simulink model "kinematic_steering"  (R2023b)
settings: Solver=VariableStepAuto  StartTime=0.0  StopTime=10.0  RelTol=1e-3
undefined symbols (not defined in the file or in its folder): static_toe_front, static_toe_rear, steering_rack_to_axis_distance
libraries: simulink_extras x7, vehdynlibsteering x1
settings Model: Creator=bglen  LastModifiedBy=bglen

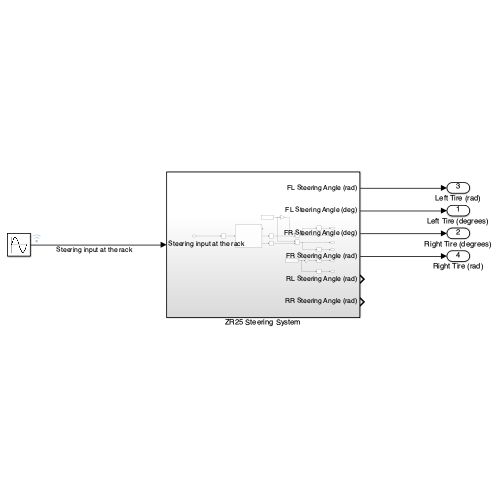
[thumbnail: Simulink's stored preview of the top-level diagram]
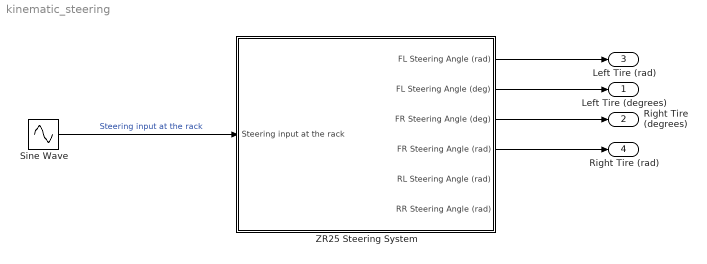
== system kinematic_steering ==
  Sine Wave : Sin  Amplitude=90  SampleTime=0
  ZR25 Steering System : Subsystem
  Left Tire (degrees) : Outport
  Right Tire (degrees) : Outport  Port=2
  Left Tire (rad) : Outport  Port=3
  Right Tire (rad) : Outport  Port=4
  wires:
  Sine Wave/1 -> ZR25 Steering System/1(Steering input at the rack)  "Steering input at the rack"
  ZR25 Steering System/1(FL Steering Angle (rad)) -> Left Tire (rad)/1
  ZR25 Steering System/2(FL Steering Angle (deg)) -> Left Tire (degrees)/1
  ZR25 Steering System/3(FR Steering Angle (deg)) -> Right Tire (degrees)/1
  ZR25 Steering System/4(FR Steering Angle (rad)) -> Right Tire (rad)/1

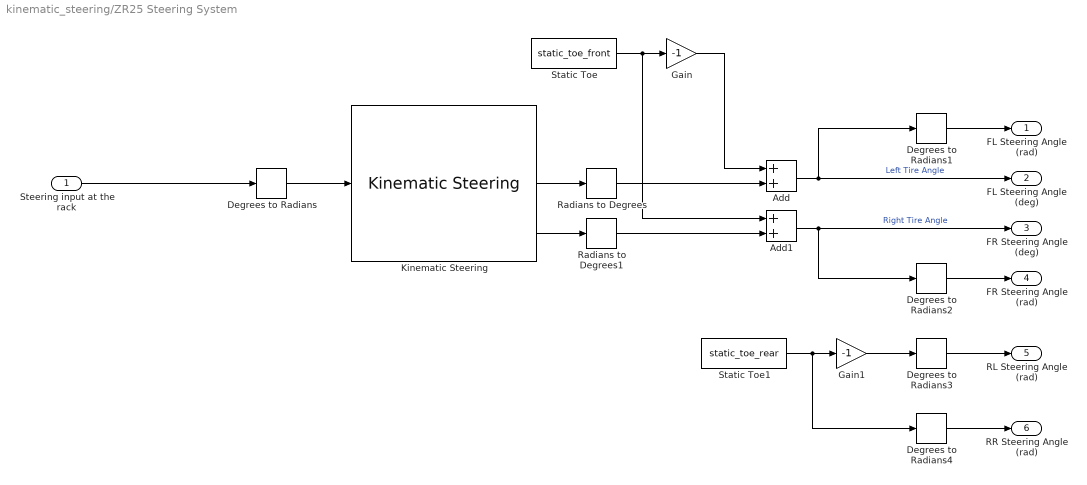
== system kinematic_steering/ZR25 Steering System ==
  Steering input at the rack : Inport
  Add : Sum
  Add1 : Sum
  Degrees to Radians{,1..4} (5 alike) : simulink_extras/Transformations/Degrees to Radians
  Gain : Gain  Gain=-1
  Gain1 : Gain  Gain=-1
  Kinematic Steering : vehdynlibsteering/Kinematic Steering  StrgType=Rack and pinion  StrgRatioType=Constant  Loc=Front  NrmlFctr=0.01  TrckWdth=track_width_front  WhlBase=1.524  Db=0  StrgRng=pi  StrgAngBpts="[-6.2832   -5.0265   -3.7699   -2.5133   -1.2566         0    1.2566    2.5133    3.7699    5.0265    6.2832]"  StrgRatioTbl=|  StrgRatio=100  PctAckIn=off  PctAck=100  PctAckTbl=ones(1,11)*100  StrgArmLngth=steering_arm_length  RckCsLngth=steering_rack_length  TieRodLngth=tie_rod_length_front  D=steering_rack_to_axis_distance  PnnRadius=steering_pinion_radius  PnnRadiusTbl="[0.0055    0.0055    0.0056    0.0057    0.0058    0.0057    0.0057    0.0057    0.0056    0.0055    0.0055]"  RodLngth=0.1  ParaArmLngth=0.9  aMode=2
      | [13.5000   13.3750   13.2500   13.1250   13.0000   13.0000   13.0000   13.1250   13.2500   13.3750   13.5000
      | ]
  Radians to Degrees : simulink_extras/Transformations/Radians to Degrees
  Radians to Degrees1 : simulink_extras/Transformations/Radians to Degrees
  Static Toe : Constant  Value=static_toe_front
  Static Toe1 : Constant  Value=static_toe_rear
  FL Steering Angle (rad) : Outport
  FL Steering Angle (deg) : Outport  Port=2
  FR Steering Angle (deg) : Outport  Port=3
  FR Steering Angle (rad) : Outport  Port=4
  RL Steering Angle (rad) : Outport  Port=5
  RR Steering Angle (rad) : Outport  Port=6
  wires:
  Degrees to Radians1/1 -> FL Steering Angle (rad)/1
  Radians to Degrees/1 -> Add/2
  Steering input at the rack/1 -> Degrees to Radians/1
  Radians to Degrees1/1 -> Add1/2
  Kinematic Steering/3 -> Radians to Degrees1/1
  Degrees to Radians2/1 -> FR Steering Angle (rad)/1
  Add1/1 -> FR Steering Angle (deg)/1, Degrees to Radians2/1  "Right Tire Angle"
  Static Toe/1 -> Add1/1, Gain/1
  Add/1 -> FL Steering Angle (deg)/1, Degrees to Radians1/1  "Left Tire Angle"
  Degrees to Radians/1 -> Kinematic Steering/1
  Gain/1 -> Add/1
  Kinematic Steering/2 -> Radians to Degrees/1
  Static Toe1/1 -> Degrees to Radians4/1, Gain1/1
  Gain1/1 -> Degrees to Radians3/1
  Degrees to Radians3/1 -> RL Steering Angle (rad)/1
  Degrees to Radians4/1 -> RR Steering Angle (rad)/1
